simulink model "reentrant_add_model"  (R2023b)
settings: Solver=FixedStepDiscrete  StartTime=0.0  StopTime=0.001  FixedStep=0.001  RelTol=1e-3
settings Model: DataDictionary=add_interface.sldd  Creator=user  LastModifiedBy=user
settings OptimizationCC: DefaultParameterBehavior=Inlined  EnhancedBackFolding=on  PassReuseOutputArgsAs=Individual arguments  OptimizeBlockOrder=speed  DifferentSizesBufferReuse=on  OptimizationCustomize=off  EfficientTunableParamExpr=on
settings DebuggingCC: ParameterTunabilityLossMsg=error
settings HardwareCC: ProdBitPerPointer=32  ProdBitPerSizeT=32  ProdBitPerPtrDiffT=32  ProdLargestAtomicInteger=Long  ProdLargestAtomicFloat=Double  ProdWordSize=32  ProdHWDeviceType=ARM Compatible->ARM Cortex  TargetLargestAtomicInteger=Long  TargetLargestAtomicFloat=Double  TargetIntDivRoundTo=Zero  TargetEndianess=LittleEndian  TargetHWDeviceType=ARM Compatible->ARM Cortex  ProdEqTarget=off
settings SFSimCC: MATLABDynamicMemAlloc=off
settings RTWCC: Description=Embedded Coder  SystemTargetFile=ert.tlc  GenCodeOnly=on  TemplateMakefile=ert_default_tmf  GenerateReport=on
settings CodeAppCC: ForceParamTrailComments=on  IgnoreCustomStorageClasses=off  OperatorAnnotations=on  SimulinkDataObjDesc=on  SFDataObjDesc=on  InsertBlockDesc=on
settings ERTTargetCC: TargetLangStandard=C99 (ISO)  CodeInterfacePackaging=Reusable function  InlinedParameterPlacement=NonHierarchical  ERTCustomFileTemplate=example_file_process.tlc

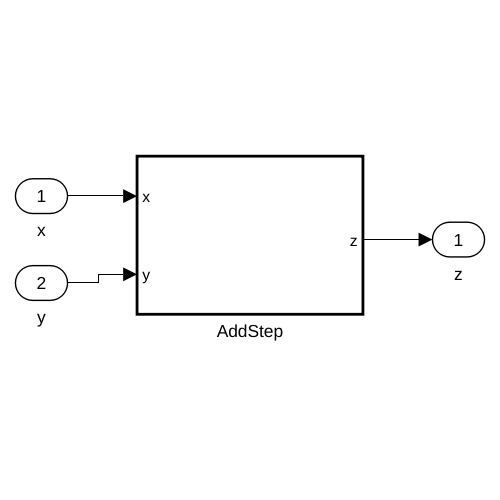
[thumbnail: Simulink's stored preview of the top-level diagram]
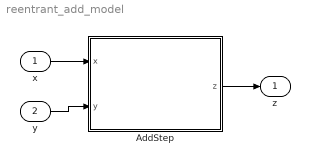
== system reentrant_add_model ==
  x : Inport  OutDataTypeStr=T_AddIn  PortDimensions=1
  y : Inport  Port=2  OutDataTypeStr=T_AddIn  PortDimensions=1
  AddStep : Subsystem  TreatAsAtomicUnit=on  RTWFcnName=AddStep  RTWFileName=AddStep
      settings: RTWFcnNameOpts=User specified  RTWFileNameOpts=User specified
  z : Outport  OutDataTypeStr=T_AddOut  PortDimensions=1
  wires:
  AddStep/1(z) -> z/1
  y/1 -> AddStep/2(y)
  x/1 -> AddStep/1(x)

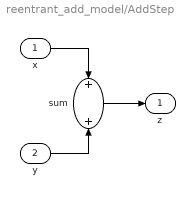
== system reentrant_add_model/AddStep ==
  x : Inport  OutDataTypeStr=T_AddIn  PortDimensions=1
  y : Inport  Port=2  OutDataTypeStr=T_AddIn  PortDimensions=1
  sum : Sum  OutDataTypeStr=T_AddOut  AccumDataTypeStr=T_AddAcc  SaturateOnIntegerOverflow=on
  z : Outport  OutDataTypeStr=T_AddOut  PortDimensions=1
  wires:
  sum/1 -> z/1
  y/1 -> sum/2
  x/1 -> sum/1
